simulink model "px4demo_Parameter_CSC_example"  (R2016a)
settings: Solver=FixedStepAuto  StartTime=0.0  StopTime=inf  FixedStep=0.5  RelTol=1e-3
InitFcn:
  | CAL_GYRO0_XSCALE = Pixhawk_CSC.Parameter( {single(1), 'CAL_GYRO0_XSCALE'}  )
  | CAL_GYRO0_YSCALE = Pixhawk_CSC.Parameter( {single(1), 'CAL_GYRO0_YSCALE'}  )
  | CAL_GYRO0_ZSCALE = Pixhawk_CSC.Parameter( {single(1), 'CAL_GYRO0_ZSCALE'}  )
  | 
  | CAL_GYRO0_XOFF = Pixhawk_CSC.Parameter( {single(0), 'CAL_GYRO0_XOFF'} )
  | CAL_GYRO0_YOFF = Pixhawk_CSC.Parameter( {single(0), 'CAL_GYRO0_YOFF'} )
  | CAL_GYRO0_ZOFF = Pixhawk_CSC.Parameter( {single(0), 'CAL_GYRO0_ZOFF'} )
libraries: pixhawk_slib_sensors_actuators x1
settings Model: SimulationMode=external  Creator=darenlee  LastModifiedBy=darenlee
settings DataIOCC: LimitDataPoints=on
settings OptimizationCC: DefaultParameterBehavior=Inlined  OptimizeModelRefInitCode=on  LifeSpan=1  MaxStackSize=64
settings DebuggingCC: AllowSymbolicDim=off
settings HardwareCC: ProdBitPerPointer=32  ProdLargestAtomicInteger=Long  ProdLargestAtomicFloat=Double  ProdWordSize=32  ProdHWDeviceType=ARM Compatible->ARM Cortex
settings ModelReferenceCC: PropagateSignalLabelsOutOfModel=off
settings RTWCC: SystemTargetFile=ert.tlc  HardwareBoard=Pixhawk PX4  TemplateMakefile=ert_default_tmf  GenerateReport=on  Toolchain=Pixhawk Toolchain  IncludeHyperlinkInReport=on  LaunchReport=on  GenerateTraceInfo=on  GenerateTraceReport=on  GenerateTraceReportSl=on  GenerateTraceReportSf=on  GenerateTraceReportEml=on
settings CodeAppCC: ForceParamTrailComments=on  IgnoreCustomStorageClasses=off  OperatorAnnotations=on  MATLABSourceComments=on
settings ERTTargetCC: ExtMode=on  ExtModeTransport=1  ExtModeMexFile=ext_serial_win32_comm  ExtModeMexArgs=1 6 115200  InlinedParameterPlacement=NonHierarchical  ERTCustomFileTemplate=PX4_codertarget_file_process.tlc  ConvertIfToSwitch=off  SuppressUnreachableDefaultCases=off

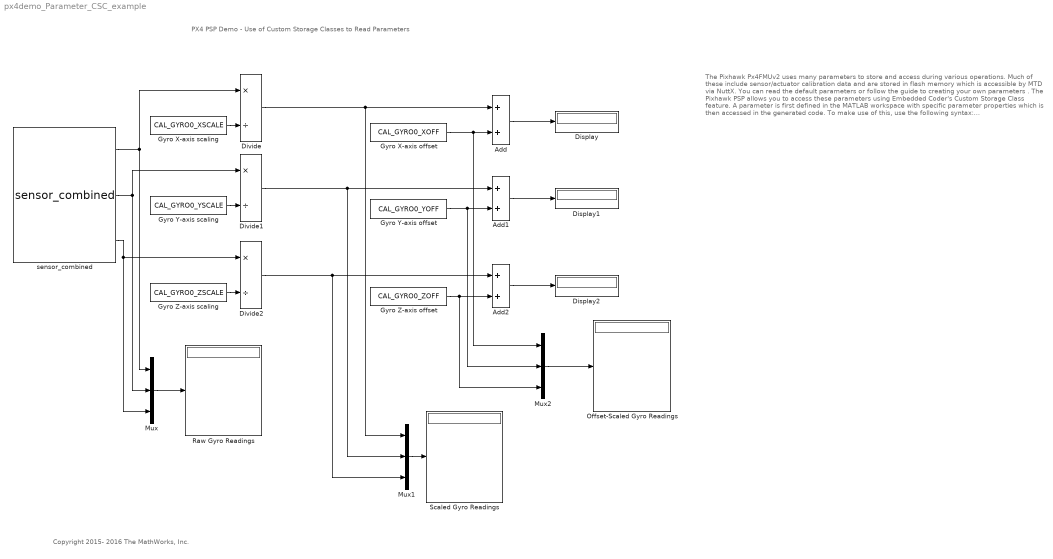
== system px4demo_Parameter_CSC_example ==
  note: PX4 PSP Demo - Use of Custom Storage Classes to Read Parameters
  note: The Pixhawk Px4FMUv2 uses many parameters to store and access during various operations.
      |
      | Much of these include sensor/actuator calibration data and are stored in flash memory which is accessible by MTD via NuttX.
      |
      | You can read the default parameters or follow the guide to creating your own parameters .
      |
      | The Pixhawk PSP allows you to access these parameters using Embedded Coder's Custom Storage Class feature.
      |
      | A parameter is first defined in the MATLAB workspace with specific parameter properties which is then accessed in the generated code.
      |
      | To make use of this, use the following syntax:
      |
      | Pixhawk_CSC.Parameter( CELL_ARRAY )
      |
      | Where CELL_ARRAY is a MATLAB cell array composed of a value (int32 or single) and a string of the parameter. For instance:
      |
      | CAL_GYRO0_XSCALE = Pixhawk_CSC.Parameter( {single(1), 'CAL_GYRO0_XSCALE'} )
      |
      | Parameters can either be int32 or single/floating precision. Please ensure you select the correct data type and the the string name matches.
      |
      | Note that for the model below, all parameters have been defined in the model's InitFcn callback function
      |
      | NOTE: This model is to be demosntrated in external mode. An alternative to being able to view these values without external mode is to modify this example to print the signals to the Nuttshell terminal using the print block
  note: Copyright 2015- 2016 The MathWorks, Inc.
  Add : Sum
  Add1 : Sum
  Add2 : Sum
  Display : Display
  Display1 : Display
  Display2 : Display
  Divide : Product  Inputs=*/
  Divide1 : Product  Inputs=*/
  Divide2 : Product  Inputs=*/
  "Gyro X-axis offset\t" : Constant  Value=CAL_GYRO0_XOFF
  Gyro X-axis scaling : Constant  Value=CAL_GYRO0_XSCALE
  Gyro Y-axis offset : Constant  Value=CAL_GYRO0_YOFF
  Gyro Y-axis scaling : Constant  Value=CAL_GYRO0_YSCALE
  Gyro Z-axis offset : Constant  Value=CAL_GYRO0_ZOFF
  Gyro Z-axis scaling : Constant  Value=CAL_GYRO0_ZSCALE
  Mux : Mux  Inputs=3
  Mux1 : Mux  Inputs=3
  Mux2 : Mux  Inputs=3
  Offset-Scaled Gyro Readings : Display
  Raw Gyro Readings : Display
  Scaled Gyro Readings : Display
  sensor_combined : pixhawk_slib_sensors_actuators/sensor_combined  sampletime=-1  show_mag=off  show_acc=off  show_gyro=on  show_baro=off  show_ts=off
  wires:
  sensor_combined/1 -> Divide/1, Mux/1
  "Gyro X-axis offset\t"/1 -> Mux2/1, Add/2
  sensor_combined/2 -> Divide1/1, Mux/2
  Gyro Y-axis offset/1 -> Mux2/2, Add1/2
  sensor_combined/3 -> Mux/3, Divide2/1
  Gyro Z-axis offset/1 -> Mux2/3, Add2/2
  Divide/1 -> Mux1/1, Add/1
  Divide1/1 -> Mux1/2, Add1/1
  Divide2/1 -> Add2/1, Mux1/3
  Add/1 -> Display/1
  Add1/1 -> Display1/1
  Add2/1 -> Display2/1
  Mux/1 -> Raw Gyro Readings/1
  Mux1/1 -> Scaled Gyro Readings/1
  Mux2/1 -> Offset-Scaled Gyro Readings/1
  Gyro X-axis scaling/1 -> Divide/2
  Gyro Y-axis scaling/1 -> Divide1/2
  Gyro Z-axis scaling/1 -> Divide2/2
